simulink model "mds_1a"  (R2014a)
settings: Solver=ode45  StartTime=0.0  StopTime=10.0  RelTol=1e-3
libraries: simulink x1
settings Model: Creator=john  LastModifiedBy=john

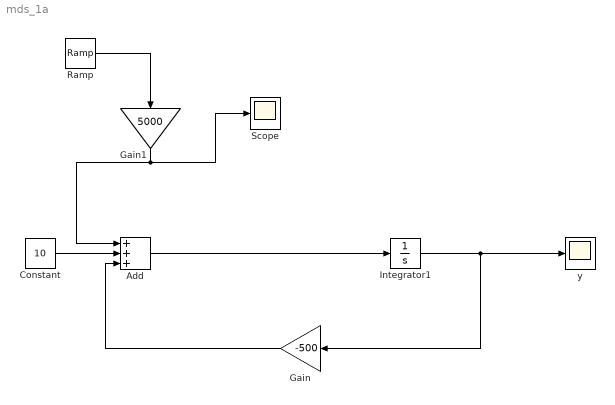
== system mds_1a ==
  Add : Sum  Inputs=+++
  Constant : Constant  Value=10
  Gain : Gain  Gain=-500
  Gain1 : Gain  Gain=5000
  Integrator1 : Integrator  InitialCondition=1
  Ramp : simulink/Sources/Ramp  slope=1  start=0  X0=0
  Scope : Scope
  y : Scope
      settings: TimeRange=50  YMin=0  YMax=2.5
  wires:
  Integrator1/1 -> Gain/1, y/1
  Gain1/1 -> Add/1, Scope/1
  Gain/1 -> Add/3
  Constant/1 -> Add/2
  Add/1 -> Integrator1/1
  Ramp/1 -> Gain1/1
